simulink model "TransmissionController"  (R2020b)
settings: Solver=VariableStepAuto  StartTime=0.0  StopTime=10.0  RelTol=1e-3
model workspace (MAT data in the model file):
  CONVERTER_DATA = [0  137.465208994  2.232; 0.1  137.065019157  2.075; 0.2  135.864449646  1.975; 0.3  135.664354728  1.846; 0.4  137.565256453  1.72; 0.5  140.366585312  1.564; 0.6  145.268910814  1.409; 0.7  152.872517717  1.254; 0.8  162.9773111  1.096; 0.81  164.27792807  1.08; 0.82  166.178829795  1.061; 0.83  167.979684062  1.043; 0.84  170.080680706  1.028; 0.85  172.781962105  1.012; 0.86  175.383196045  1.002; 0.87  179.585189333  1.002; 0.88  183.587087703  1.001; 0.89  189.890077635  0.998; 0.9  197.693779455  0.999; 0.92  215.902417037  1.001; 0.94  244.515990379  1.002]
  VEHICLE_DATA = [3.23; 40; 0.02; 1; 12.0941478573; 0]
undefined symbols (not defined in the file): emap, Iei, ne_vec, th_vec
settings Model: OrderedModelArguments=off  Creator=shivanshu shukla  LastModifiedBy=shivanshu shukla

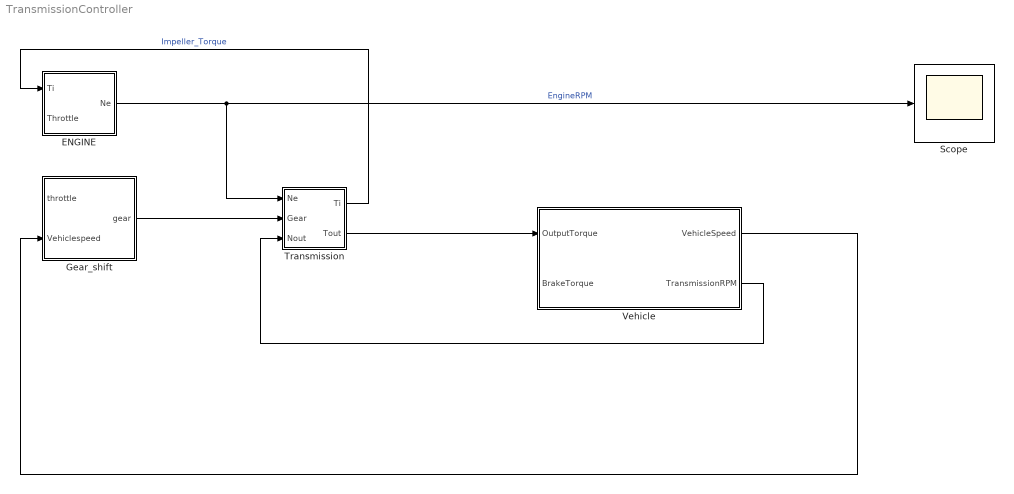
== system TransmissionController ==
  ENGINE : Subsystem
  Gear_shift : Stateflow chart  TreatAsAtomicUnit=on
  Scope : Scope  NumInputPorts=3
  Transmission : Subsystem
  Vehicle : Subsystem  mask{Rfd=VEHICLE_DATA(1), rload0=VEHICLE_DATA(2), rload2=VEHICLE_DATA(3), Rw=VEHICLE_DATA(4), Iv=VEHICLE_DATA(5), N20=VEHICLE_DATA(6)/VEHICLE_DATA(4)*VEHICLE_DATA(1)}
      mask prompts: Rfd "final drive ratio"; rload0 "drag friction at wheels"; rload2 "aerodynamic drag"; Rw "wheel radius"; Iv "vehicle inertia"; N20 "initial transmission output speed"
  wires:
  ENGINE/1(Ne) -> Transmission/1(Ne), Scope/2  "EngineRPM"
  Gear_shift/1(gear) -> Transmission/2(Gear)
  Transmission/1(Ti) -> ENGINE/1(Ti)  "Impeller_Torque"
  Transmission/2(Tout) -> Vehicle/1(OutputTorque)
  Vehicle/2(TransmissionRPM) -> Transmission/3(Nout)
  Vehicle/1(VehicleSpeed) -> Gear_shift/2(Vehiclespeed)

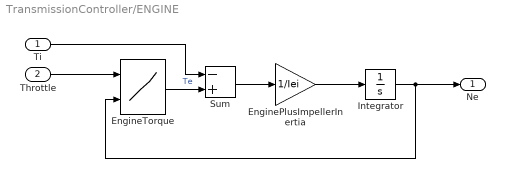
== system TransmissionController/ENGINE ==
  Ti : Inport  Unit=ft*lbf@torque
  Throttle : Inport  Port=2  Unit=%
  EnginePlusImpellerInertia : Gain  Gain=1/Iei  SaturateOnIntegerOverflow=on  OutDataTypeStr=Inherit: Same as input  ParamDataTypeStr=Inherit: Same as input
  EngineTorque : Lookup_n-D  BreakpointsForDimension1=th_vec  BreakpointsForDimension2=ne_vec  Table=emap  InputSameDT=on
      settings: InputPortMap=u0,u1
  Integrator : Integrator
  Sum : Sum  Inputs=-+  InputSameDT=on  SaturateOnIntegerOverflow=on  OutDataTypeStr=Inherit: Same as first input
  Ne : Outport  Unit=rpm  VectorParamsAs1DForOutWhenUnconnected=off
  wires:
  Integrator/1 -> Ne/1, EngineTorque/2
  Sum/1 -> EnginePlusImpellerInertia/1
  Ti/1 -> Sum/1
  EnginePlusImpellerInertia/1 -> Integrator/1
  Throttle/1 -> EngineTorque/1
  EngineTorque/1 -> Sum/2  "Te"

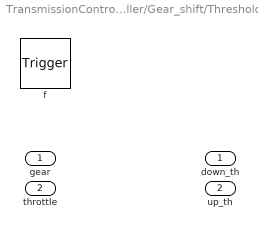
== system TransmissionController/Gear_shift/ThresholdCal ==
  gear : Inport  OutDataTypeStr=double  PortDimensions=1
  throttle : Inport  Port=2  OutDataTypeStr=double  PortDimensions=1
  f : TriggerPort  TriggerType=function-call  VariantControl=(inherit)
      settings: CopyFcn=Stateflow.SLINSF.SimulinkMan.removeBlockPreDeleteFcn  PreDeleteFcn=Stateflow.SLINSF.SimulinkMan.unsafePredeleteFcn
  down_th : Outport
  up_th : Outport  Port=2

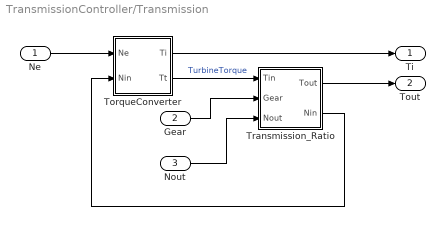
== system TransmissionController/Transmission ==
  Ne : Inport
  Gear : Inport  Port=2
  Nout : Inport  Port=3
  TorqueConverter : Subsystem  mask(torque converter){speedratio=CONVERTER_DATA(:,1), Kfactor=CONVERTER_DATA(:,2), Torkratio=CONVERTER_DATA(:,3)}
      mask prompts: speedratio "speed ratio"; Kfactor "K factor"; Torkratio "torque ratio"
      mask help: torque converter
      mask Help: Torque converter input and output torques are computed as a function of the input and output speeds
      mask Display: plot([cos([90:10:450]*pi/180),.63*cos([90:10:450]*pi/180),.63*cos([90:10:240]*pi/180),cos([240:10:300]*pi/180),.63*cos([300]*pi/180)],[sin([90:10:450]*pi/180),.63*sin([90:10:450]*pi/180)+.1,.63*sin([90:10:240]*pi/180)+.1,sin([240:10:300]*pi/180),.63*sin([300]*pi/180)+.1])
  Transmission_Ratio : Subsystem
  Ti : Outport
  Tout : Outport  Port=2
  wires:
  Transmission_Ratio/1(Tout) -> Tout/1
  TorqueConverter/2(Tt) -> Transmission_Ratio/1(Tin)  "TurbineTorque"
  TorqueConverter/1(Ti) -> Ti/1
  Gear/1 -> Transmission_Ratio/2(Gear)
  Ne/1 -> TorqueConverter/1(Ne)
  Transmission_Ratio/2(Nin) -> TorqueConverter/2(Nin)
  Nout/1 -> Transmission_Ratio/3(Nout)

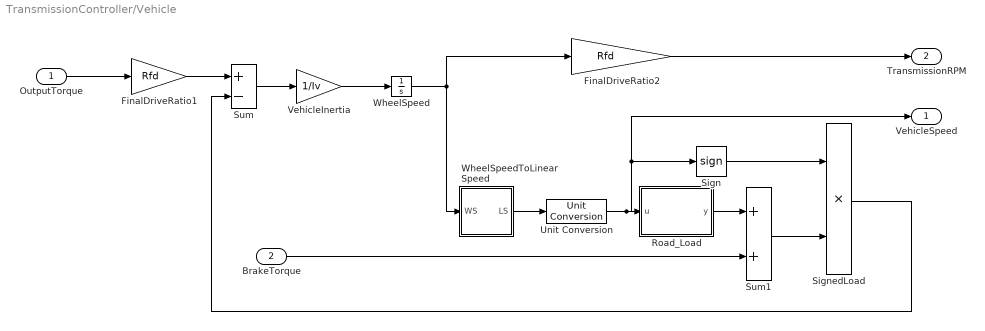
== system TransmissionController/Vehicle ==
  OutputTorque : Inport  Unit=ft*lbf@torque
  BrakeTorque : Inport  Port=2  Unit=ft*lbf@torque
  FinalDriveRatio1 : Gain  Gain=Rfd  SaturateOnIntegerOverflow=on  OutDataTypeStr=Inherit: Same as input  ParamDataTypeStr=Inherit: Same as input
  FinalDriveRatio2 : Gain  Gain=Rfd  SaturateOnIntegerOverflow=on  OutDataTypeStr=Inherit: Same as input  ParamDataTypeStr=Inherit: Same as input
  Road_Load : MATLAB Function  TreatAsAtomicUnit=on
  Sign : Signum
  SignedLoad : Product  InputSameDT=on  SaturateOnIntegerOverflow=on  OutDataTypeStr=Inherit: Same as first input
  Sum : Sum  Inputs=+-  InputSameDT=on  SaturateOnIntegerOverflow=on  OutDataTypeStr=Inherit: Same as first input
  Sum1 : Sum  InputSameDT=on  SaturateOnIntegerOverflow=on  OutDataTypeStr=Inherit: Same as first input
  Unit Conversion : UnitConversion
  VehicleInertia : Gain  Gain=1/Iv  SaturateOnIntegerOverflow=on  OutDataTypeStr=Inherit: Same as input  ParamDataTypeStr=Inherit: Same as input
  WheelSpeed : Integrator  InitialCondition=N20/Rfd  ZeroCross=off
  WheelSpeedToLinearSpeed : Subsystem
  VehicleSpeed : Outport  Unit=mph  VectorParamsAs1DForOutWhenUnconnected=off
  TransmissionRPM : Outport  Port=2  Unit=rpm  VectorParamsAs1DForOutWhenUnconnected=off
  wires:
  OutputTorque/1 -> FinalDriveRatio1/1
  FinalDriveRatio2/1 -> TransmissionRPM/1
  Sum1/1 -> SignedLoad/2
  Unit Conversion/1 -> VehicleSpeed/1, Sign/1, Road_Load/1(u)
  VehicleInertia/1 -> WheelSpeed/1
  BrakeTorque/1 -> Sum1/2
  SignedLoad/1 -> Sum/2
  Sum/1 -> VehicleInertia/1
  Sign/1 -> SignedLoad/1
  WheelSpeed/1 -> WheelSpeedToLinearSpeed/1(WS), FinalDriveRatio2/1
  FinalDriveRatio1/1 -> Sum/1
  WheelSpeedToLinearSpeed/1(LS) -> Unit Conversion/1
  Road_Load/1(y) -> Sum1/1

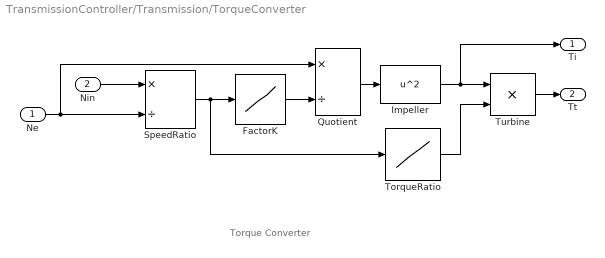
== system TransmissionController/Transmission/TorqueConverter ==
  note: Torque Converter
  Ne : Inport
  Nin : Inport  Port=2
  FactorK : Lookup_n-D  NumberOfTableDimensions=1  BreakpointsForDimension1=speedratio  Table=Kfactor  SaturateOnIntegerOverflow=on  InputSameDT=on
  Impeller : Fcn  Expr=u^2
  Quotient : Product  Inputs=*/  InputSameDT=on  SaturateOnIntegerOverflow=on  OutDataTypeStr=Inherit: Same as first input
  SpeedRatio : Product  Inputs=*/  InputSameDT=on  SaturateOnIntegerOverflow=on  OutDataTypeStr=Inherit: Same as first input
  TorqueRatio : Lookup_n-D  NumberOfTableDimensions=1  BreakpointsForDimension1=speedratio  Table=Torkratio  SaturateOnIntegerOverflow=on  InputSameDT=on
  Turbine : Product  InputSameDT=on  SaturateOnIntegerOverflow=on  OutDataTypeStr=Inherit: Same as first input
  Ti : Outport  VectorParamsAs1DForOutWhenUnconnected=off
  Tt : Outport  Port=2  VectorParamsAs1DForOutWhenUnconnected=off
  wires:
  TorqueRatio/1 -> Turbine/2
  Quotient/1 -> Impeller/1
  FactorK/1 -> Quotient/2
  SpeedRatio/1 -> TorqueRatio/1, FactorK/1
  Impeller/1 -> Turbine/1, Ti/1
  Turbine/1 -> Tt/1
  Ne/1 -> SpeedRatio/2, Quotient/1
  Nin/1 -> SpeedRatio/1

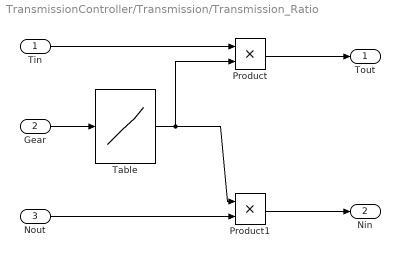
== system TransmissionController/Transmission/Transmission_Ratio ==
  Tin : Inport  Unit=ft*lbf@torque
  Gear : Inport  Port=2  Unit=1
  Nout : Inport  Port=3  Unit=rpm
  Product : Product  InputSameDT=on  SaturateOnIntegerOverflow=on  OutDataTypeStr=Inherit: Same as first input
  Product1 : Product  InputSameDT=on  SaturateOnIntegerOverflow=on  OutDataTypeStr=Inherit: Same as first input
  Table : Lookup_n-D  NumberOfTableDimensions=1  BreakpointsForDimension1=[1 2 3 4]  Table=[2.393 1.450 1.000 0.677]  OutDataTypeStr=double  SaturateOnIntegerOverflow=on  InputSameDT=on  LockScale=on
  Tout : Outport  Unit=ft*lbf@torque  VectorParamsAs1DForOutWhenUnconnected=off
  Nin : Outport  Port=2  Unit=rpm  VectorParamsAs1DForOutWhenUnconnected=off
  wires:
  Gear/1 -> Table/1
  Product1/1 -> Nin/1
  Table/1 -> Product1/1, Product/2
  Nout/1 -> Product1/2
  Tin/1 -> Product/1
  Product/1 -> Tout/1

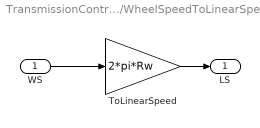
== system TransmissionController/Vehicle/WheelSpeedToLinearSpeed ==
  WS : Inport  Unit=rpm
  ToLinearSpeed : Gain  Gain=2*pi*Rw  SaturateOnIntegerOverflow=on  OutDataTypeStr=Inherit: Same as input  ParamDataTypeStr=Inherit: Same as input
  LS : Outport  Unit=ft/min  VectorParamsAs1DForOutWhenUnconnected=off
  wires:
  ToLinearSpeed/1 -> LS/1
  WS/1 -> ToLinearSpeed/1

== matlab function TransmissionController/Vehicle/Road_Load ==
  data: u input; y output
function y = fcn(u)

y = rload0 + rload2*u^2;

== stateflow chart TransmissionController/Gear_shift ==
  state Gear_State [parallel]
    settings: executionOrder=1
    state Gear1
      en:
      gear=1;
    state Gear2
      en:
      gear=2;
    state Gear3
      en:
      gear=3;
    state Gear4
      en:
      gear=4;
    (default) -> Gear1
    Gear1 -> Gear2 : up
    Gear2 -> Gear3 [order 1] : up
    Gear3 -> Gear4 [order 1] : up
    Gear2 -> Gear1 [order 2] : down
    Gear3 -> Gear2 [order 2] : down
    Gear4 -> Gear3 : down
  state Selection_State [parallel]
    du:
    [down_th,up_th]=ThresholdCal(gear,throttle);
    settings: executionOrder=2
    state Steady_state
    state Downshift
    state UpShift
    (default) -> Steady_state
    Steady_state -> UpShift [order 1] : [Vehiclespeed>up_th]
    Steady_state -> Downshift [order 2] : [Vehiclespeed<down_th]
    Downshift -> Steady_state [order 1] : after(2,tick)
        | [Vehiclespeed<=down_th]
        | {Gear_State.down}
    Downshift -> Steady_state [order 2] : [Vehiclespeed>down_th]
    UpShift -> Steady_state [order 2] : [Vehiclespeed>up_th]
    UpShift -> Steady_state [order 1] : after(2,tick)
        | [Vehiclespeed>=up_th]
        | {Gear_State.up}
  state [down_th,up_th]=ThresholdCal(gear,throttle) [function]
  data: down_th function_output; up_th function_output; gear function_input double size=1; throttle function_input double size=1; gear output; up_th local; down_th local; throttle input; Vehiclespeed input
  events: up local FUNCTION_CALL_EVENT; down local FUNCTION_CALL_EVENT
